simulink model "dfig_group_6_backsave"  (R2019b)
settings: Solver=ode23t  StartTime=0.0  StopTime=100  RelTol=1e-3
undefined symbols (not defined in the file): i, j
libraries: eeGeneralControl x2
settings Model: SimulationMode=accelerator  Creator=aspar  LastModifiedBy=aspar
settings DebuggingCC: UnconnectedInputMsg=none  UnconnectedOutputMsg=none  UnconnectedLineMsg=none
settings ModelReferenceCC: EnableRefExpFcnMdlSchedulingChecks=off
settings RTWCC: Description=Generic Real-Time Target

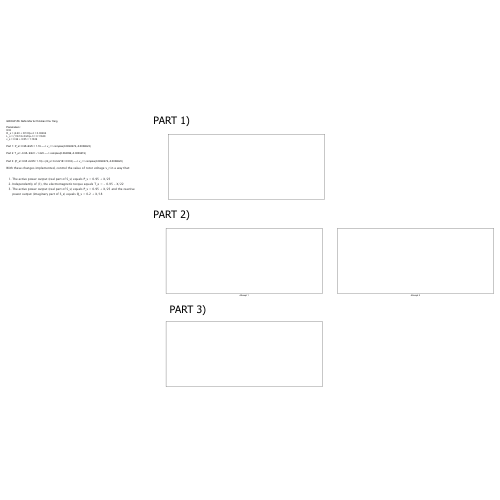
[thumbnail: Simulink's stored preview of the top-level diagram]
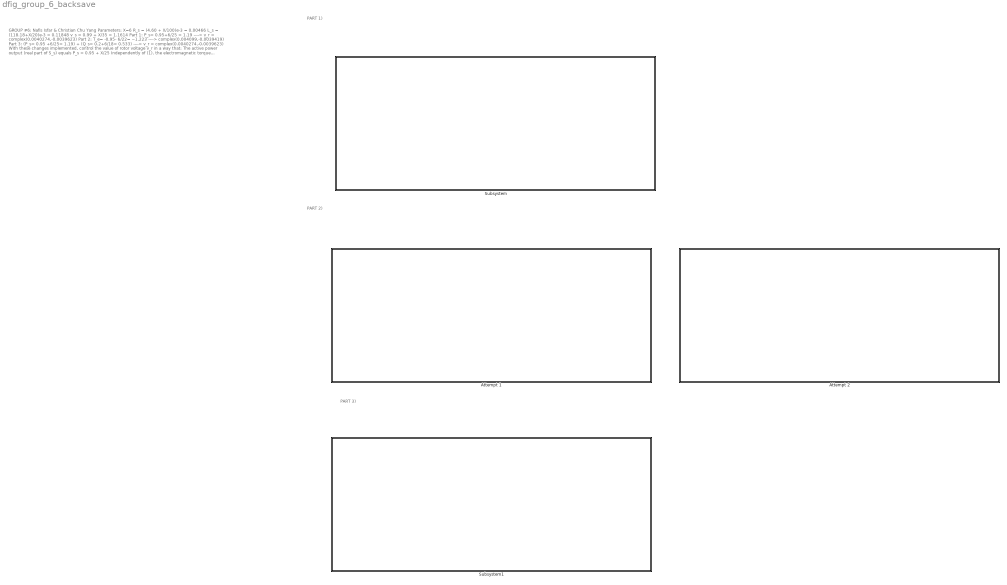
== system dfig_group_6_backsave ==
  note: GROUP #6: Nafis Isfar & Christian Chu Yang
      |
      | Parameters:
      | X=6
      | R_s = (4.60 + X/100)e-3 = 0.00466
      | L_s = (118.18+X/20)e-3 = 0.11848
      | v_s = 0.99 + X/35 = 1.1614
      | Part 1: P_s= 0.95+6/25 = 1.19 ----> v_r = complex(0.0040274,-0.0039623)
      | Part 2: T_e= -0.95- 6/22= −1.223 ----> complex(0.004099,-0.0039419)
      | Part 3: (P_s= 0.95 +6/25= 1.19) + (Q_s= 0.2+6/18= 0.533) ----> v_r = complex(0.0040274,-0.0039623)
      |
      | With these changes implemented, control the value of rotor voltage v_r in a way that:
      | The active power output (real part of S_s) equals P_s = 0.95 + X/25
      | Independently of (1), the electromagnetic torque equals T_e = - 0.95 - X/22
      | The active power output (real part of S_s) equals P_s = 0.95 + X/25 and the reactive power output (imaginary part of S_s) equals Q_s = 0.2 + X/18
  note: PART 1)
  note: PART 2)
  note: PART 3)
  Attempt 1 : Subsystem
  Attempt 2 : Subsystem
  Subsystem : Subsystem
  Subsystem1 : Subsystem

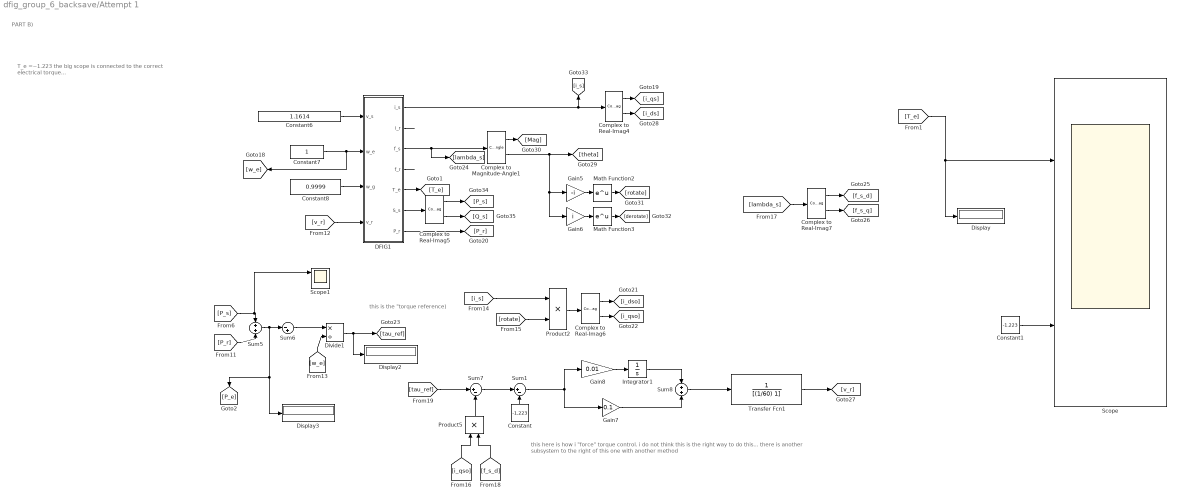
== system dfig_group_6_backsave/Attempt 1 ==
  note: this here is how i "force" torque control. i do not think this is the right way to do this... there is another subsystem to the right of this one with another method
  note: T_e =−1.223
      | the big scope is connected to the correct electrical torque...
  note: this is the "torque reference)
  note: PART B)
  Complex to Magnitude-Angle1 : ComplexToMagnitudeAngle
  Complex to Real-Imag{4..7} (4 alike) : ComplexToRealImag
  Constant : Constant  Value=-1.223
  Constant1 : Constant  Value=-1.223
  Constant6 : Constant  Value=1.1614
  Constant7 : Constant
  Constant8 : Constant  Value=0.9999
  DFIG1 : Subsystem  mask{R_s=4.66e-3, R_r=3.8e-3, L_m=1.99, L_s=118.48e-3}
  Display : Display
  Display2 : Display
  Display3 : Display
  Divide1 : Product  Inputs=*/
  Gain5 : Gain  Gain=-i
  Gain6 : Gain  Gain=i
  Gain7 : Gain  Gain=0.1
  Gain8 : Gain  Gain=0.01
  Integrator1 : Integrator
  Math Function2 : Math  SaturateOnIntegerOverflow=on
  Math Function3 : Math  SaturateOnIntegerOverflow=on
  Product2 : Product
  Product5 : Product
  Scope : Scope  NumInputPorts=2
  Scope1 : Scope  NumInputPorts=3
  Sum1 : Sum  Inputs=|+-
  Sum5 : Sum  Inputs=+|+
  Sum6 : Sum  Inputs=|-+
  Sum7 : Sum  Inputs=|+-
  Sum8 : Sum  Inputs=+|+
  Transfer Fcn1 : TransferFcn  Denominator=[(1/60) 1]
  wires:
  DFIG1/3(f_s) -> Complex to Magnitude-Angle1/1, [lambda_s]
  DFIG1/1(i_s) -> Complex to Real-Imag4/1, [i_s]
  [P_s] -> Sum5/1, Scope1/1
  Sum1/1 -> Gain7/1, Gain8/1
  Transfer Fcn1/1 -> [v_r]
  Sum6/1 -> Divide1/1
  [rotate] -> Product2/2
  Sum8/1 -> Transfer Fcn1/1
  DFIG1/4(f_r) -> ?
  Complex to Magnitude-Angle1/2 -> [theta], Gain5/1, Gain6/1
  Gain7/1 -> Sum8/2
  [i_qso] -> Product5/1
  DFIG1/7(P_r) -> [P_r]
  Gain8/1 -> Integrator1/1
  [f_s_d] -> Product5/2
  Complex to Real-Imag6/2 -> [i_qso]
  Math Function3/1 -> [derotate]
  Divide1/1 -> [tau_ref], Display2/1
  [tau_ref] -> Sum7/1
  Complex to Real-Imag7/1 -> [f_s_d]
  Constant6/1 -> DFIG1/1(v_s)
  [lambda_s] -> Complex to Real-Imag7/1
  Gain6/1 -> Math Function3/1
  Complex to Real-Imag4/2 -> [i_ds]
  [i_s] -> Product2/1
  [w_e] -> Divide1/2
  Complex to Real-Imag5/1 -> [P_s]
  Complex to Real-Imag7/2 -> [f_s_q]
  Product5/1 -> Sum7/2
  Product2/1 -> Complex to Real-Imag6/1
  Complex to Real-Imag6/1 -> [i_dso]
  Integrator1/1 -> Sum8/1
  Gain5/1 -> Math Function2/1
  Sum5/1 -> [P_e], Display3/1, Sum6/1
  DFIG1/6(S_s) -> Complex to Real-Imag5/1
  Math Function2/1 -> [rotate]
  Complex to Real-Imag5/2 -> [Q_s]
  Complex to Real-Imag4/1 -> [i_qs]
  Constant8/1 -> DFIG1/3(w_g)
  Complex to Magnitude-Angle1/1 -> [Mag]
  Constant7/1 -> [w_e], DFIG1/2(w_e)
  [v_r] -> DFIG1/4(v_r)
  DFIG1/2(i_r) -> ?
  [P_r] -> Sum5/2
  DFIG1/5(T_e) -> [T_e]
  [T_e] -> Display/1, Scope/1
  Sum7/1 -> Sum1/1
  Constant/1 -> Sum1/2
  Constant1/1 -> Scope/2

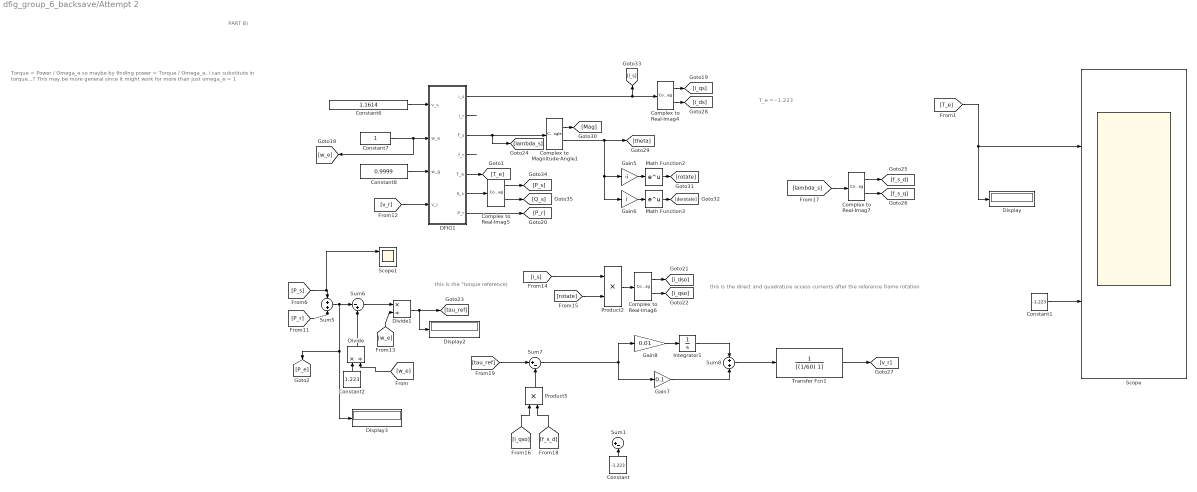
== system dfig_group_6_backsave/Attempt 2 ==
  note: Torque = Power / Omega_e
      | so maybe by finding power = Torque / Omega_e, i can substitute in torque...?
      | This may be more general since it might work for more than just omega_e = 1
  note: T_e =−1.223
  note: this is the direct and quadrature access currents after the reference frame rotation
  note: this is the "torque reference)
  note: PART B)
  Complex to Magnitude-Angle1 : ComplexToMagnitudeAngle
  Complex to Real-Imag{4..7} (4 alike) : ComplexToRealImag
  Constant : Constant  Value=-1.223
  Constant1 : Constant  Value=-1.223
  Constant2 : Constant  Value=1.223
  Constant6 : Constant  Value=1.1614
  Constant7 : Constant
  Constant8 : Constant  Value=0.9999
  DFIG1 : Subsystem  mask{R_s=4.66e-3, R_r=3.8e-3, L_m=1.99, L_s=118.48e-3}
  Display : Display
  Display2 : Display
  Display3 : Display
  Divide : Product  Inputs=*/
  Divide1 : Product  Inputs=*/
  Gain5 : Gain  Gain=-i
  Gain6 : Gain  Gain=i
  Gain7 : Gain  Gain=0.1
  Gain8 : Gain  Gain=0.01
  Integrator1 : Integrator
  Math Function2 : Math  SaturateOnIntegerOverflow=on
  Math Function3 : Math  SaturateOnIntegerOverflow=on
  Product2 : Product
  Product5 : Product
  Scope : Scope  NumInputPorts=2
  Scope1 : Scope  NumInputPorts=3
  Sum1 : Sum  Inputs=|+-
  Sum5 : Sum  Inputs=+|+
  Sum6 : Sum  Inputs=|-+
  Sum7 : Sum  Inputs=|+-
  Sum8 : Sum  Inputs=+|+
  Transfer Fcn1 : TransferFcn  Denominator=[(1/60) 1]
  wires:
  DFIG1/3(f_s) -> Complex to Magnitude-Angle1/1, [lambda_s]
  DFIG1/1(i_s) -> Complex to Real-Imag4/1, [i_s]
  [P_s] -> Sum5/1, Scope1/1
  Sum7/1 -> Gain7/1, Gain8/1
  Transfer Fcn1/1 -> [v_r]
  Sum6/1 -> Divide1/1
  [rotate] -> Product2/2
  Sum8/1 -> Transfer Fcn1/1
  DFIG1/4(f_r) -> ?
  Complex to Magnitude-Angle1/2 -> [theta], Gain5/1, Gain6/1
  Gain7/1 -> Sum8/2
  [i_qso] -> Product5/1
  DFIG1/7(P_r) -> [P_r]
  Gain8/1 -> Integrator1/1
  [f_s_d] -> Product5/2
  Complex to Real-Imag6/2 -> [i_qso]
  Math Function3/1 -> [derotate]
  Divide1/1 -> [tau_ref], Display2/1
  [tau_ref] -> Sum7/1
  Complex to Real-Imag7/1 -> [f_s_d]
  Constant6/1 -> DFIG1/1(v_s)
  [lambda_s] -> Complex to Real-Imag7/1
  Gain6/1 -> Math Function3/1
  Complex to Real-Imag4/2 -> [i_ds]
  [i_s] -> Product2/1
  [w_e] -> Divide1/2
  Complex to Real-Imag5/1 -> [P_s]
  Complex to Real-Imag7/2 -> [f_s_q]
  Product5/1 -> Sum7/2
  Product2/1 -> Complex to Real-Imag6/1
  Complex to Real-Imag6/1 -> [i_dso]
  Integrator1/1 -> Sum8/1
  Gain5/1 -> Math Function2/1
  Sum5/1 -> [P_e], Display3/1, Sum6/1
  DFIG1/6(S_s) -> Complex to Real-Imag5/1
  Math Function2/1 -> [rotate]
  Complex to Real-Imag5/2 -> [Q_s]
  Complex to Real-Imag4/1 -> [i_qs]
  Constant8/1 -> DFIG1/3(w_g)
  Complex to Magnitude-Angle1/1 -> [Mag]
  Constant7/1 -> [w_e], DFIG1/2(w_e)
  [v_r] -> DFIG1/4(v_r)
  DFIG1/2(i_r) -> ?
  [P_r] -> Sum5/2
  DFIG1/5(T_e) -> [T_e]
  [T_e] -> Display/1, Scope/1
  Constant1/1 -> Scope/2
  Constant/1 -> Sum1/2
  Divide/1 -> Sum6/2
  Constant2/1 -> Divide/1
  [w_e] -> Divide/2

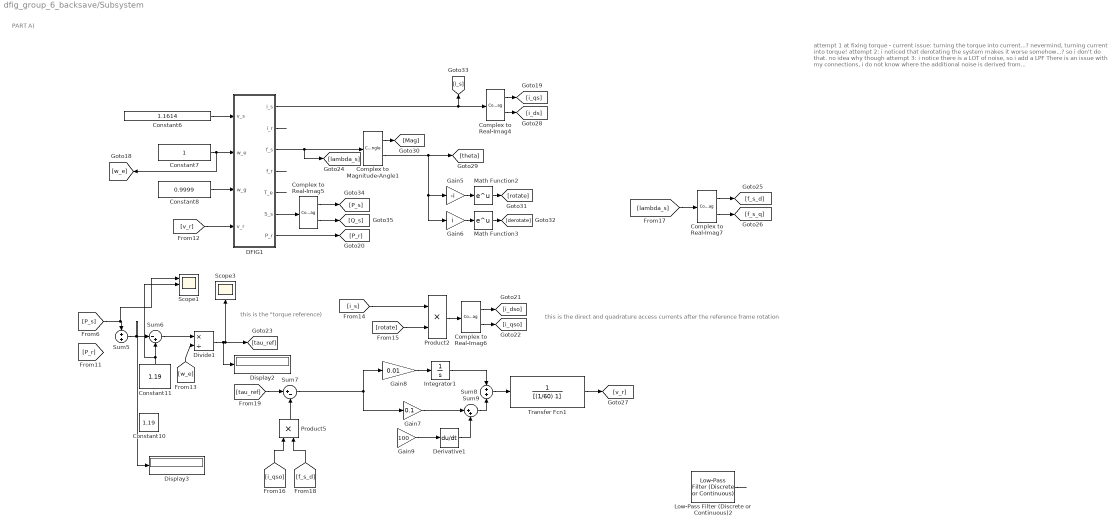
== system dfig_group_6_backsave/Subsystem ==
  note: this is the direct and quadrature access currents after the reference frame rotation
  note: attempt 1 at fixing torque - current issue: turning the torque into current...? nevermind, turning current into torque!
      |
      | attempt 2: i noticed that derotating the system makes it worse somehow...? so i don't do that. no idea why though
      |
      | attempt 3: i notice there is a LOT of noise, so i add a LPF
      |
      | There is an issue with my connections, i do not know where the additional noise is derived from...
  note: this is the "torque reference)
  note: PART A)
  Complex to Magnitude-Angle1 : ComplexToMagnitudeAngle
  Complex to Real-Imag{4..7} (4 alike) : ComplexToRealImag
  Constant10 : Constant  Value=1.19
  Constant11 : Constant  Value=1.19
  Constant6 : Constant  Value=1.1614
  Constant7 : Constant
  Constant8 : Constant  Value=0.9999
  DFIG1 : Subsystem  mask{R_s=4.66e-3, R_r=3.8e-3, L_m=1.99, L_s=118.48e-3}
  Derivative1 : Derivative
  Display2 : Display
  Display3 : Display
  Divide1 : Product  Inputs=*/
  Gain5 : Gain  Gain=-i
  Gain6 : Gain  Gain=i
  Gain7 : Gain  Gain=0.1
  Gain8 : Gain  Gain=0.01
  Gain9 : Gain  Gain=100
  Integrator1 : Integrator
  Low-Pass Filter (Discrete or Continuous)2 : eeGeneralControl/Low-Pass Filter (Discrete or Continuous)  K=1  T=1/60  B=inf  A=-inf  init_option=Inherited from block input  x0=0  Ts=-1
  Math Function2 : Math  SaturateOnIntegerOverflow=on
  Math Function3 : Math  SaturateOnIntegerOverflow=on
  Product2 : Product
  Product5 : Product
  Scope1 : Scope  NumInputPorts=3
  Scope3 : Scope
  Sum5 : Sum  Inputs=+|+
  Sum6 : Sum  Inputs=|-+
  Sum7 : Sum  Inputs=|+-
  Sum8 : Sum  Inputs=+|+
  Sum9 : Sum  Inputs=|++
  Transfer Fcn1 : TransferFcn  Denominator=[(1/60) 1]
  wires:
  DFIG1/3(f_s) -> Complex to Magnitude-Angle1/1, [lambda_s]
  DFIG1/1(i_s) -> Complex to Real-Imag4/1, [i_s]
  [P_s] -> Sum5/1, Scope1/1
  Gain9/1 -> Derivative1/1
  Sum7/1 -> Gain7/1, Gain8/1
  Transfer Fcn1/1 -> [v_r]
  Gain7/1 -> Sum9/1
  Sum6/1 -> Divide1/1
  [rotate] -> Product2/2
  Sum8/1 -> Transfer Fcn1/1
  DFIG1/4(f_r) -> ?
  Complex to Magnitude-Angle1/2 -> [theta], Gain5/1, Gain6/1
  Sum9/1 -> Sum8/2
  Derivative1/1 -> Sum9/2
  [i_qso] -> Product5/1
  DFIG1/7(P_r) -> [P_r]
  Gain8/1 -> Integrator1/1
  ? -> Gain9/1
  [f_s_d] -> Product5/2
  Complex to Real-Imag6/2 -> [i_qso]
  Math Function3/1 -> [derotate]
  DFIG1/5(T_e) -> ?
  Divide1/1 -> [tau_ref], Scope3/1, Display2/1
  [tau_ref] -> Sum7/1
  Constant11/1 -> Sum6/2, Scope1/2
  Complex to Real-Imag7/1 -> [f_s_d]
  Constant6/1 -> DFIG1/1(v_s)
  [lambda_s] -> Complex to Real-Imag7/1
  Gain6/1 -> Math Function3/1
  ? -> Low-Pass Filter (Discrete or Continuous)2/1
  Complex to Real-Imag4/2 -> [i_ds]
  [i_s] -> Product2/1
  [w_e] -> Divide1/2
  Complex to Real-Imag5/1 -> [P_s]
  Complex to Real-Imag7/2 -> [f_s_q]
  Product5/1 -> Sum7/2
  Product2/1 -> Complex to Real-Imag6/1
  Complex to Real-Imag6/1 -> [i_dso]
  Integrator1/1 -> Sum8/1
  Gain5/1 -> Math Function2/1
  Sum5/1 -> Sum6/1, Display3/1
  DFIG1/6(S_s) -> Complex to Real-Imag5/1
  Math Function2/1 -> [rotate]
  Complex to Real-Imag5/2 -> [Q_s]
  Complex to Real-Imag4/1 -> [i_qs]
  Constant8/1 -> DFIG1/3(w_g)
  Complex to Magnitude-Angle1/1 -> [Mag]
  Constant7/1 -> DFIG1/2(w_e), [w_e]
  [v_r] -> DFIG1/4(v_r)
  DFIG1/2(i_r) -> ?
  Low-Pass Filter (Discrete or Continuous)2/1 -> ?

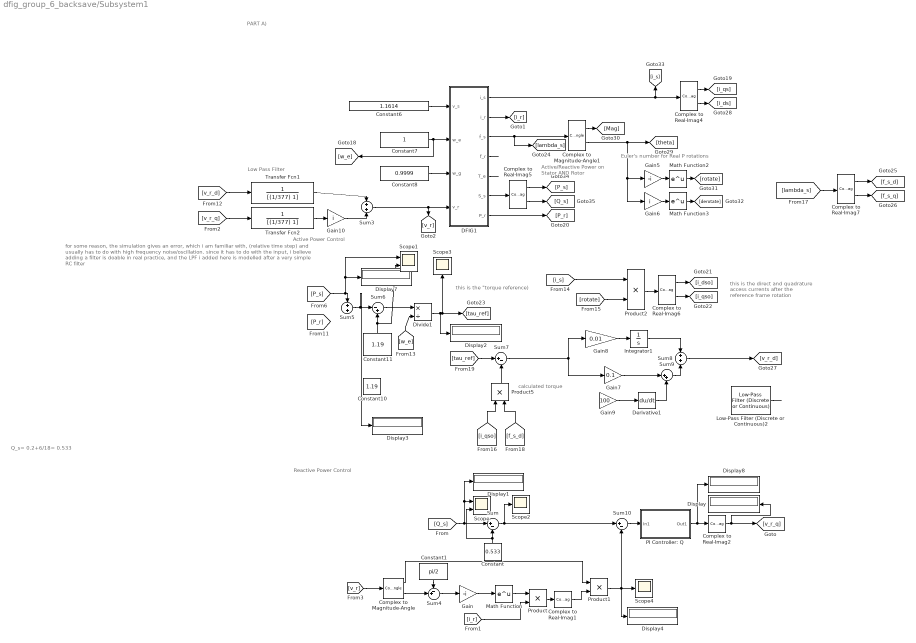
== system dfig_group_6_backsave/Subsystem1 ==
  note: calculated torque
  note: Euler's number for Real P rotations
  note: Active/Reactive
      | Power on
      | Stator AND Rotor
  note: Reactive Power Control
  note: Low Pass Filter
  note: for some reason, the simulation gives an error,
      | which i am familiar with, (relative time step)
      | and usually has to do with high frequency
      | noise/oscillation. since it has to do with the input,
      | i believe adding a filter is doable in real practice,
      | and the LPF i added here is modelled after a
      | very simple RC filter
  note: Q_s= 0.2+6/18= 0.533
  note: Active Power
      | Control
  note: this is the direct and quadrature access currents after the reference frame rotation
  note: this is the "torque reference)
  note: PART A)
  Complex to Magnitude-Angle : ComplexToMagnitudeAngle
  Complex to Magnitude-Angle1 : ComplexToMagnitudeAngle
  Complex to Real-Imag1 : ComplexToRealImag  Output=Real
  Complex to Real-Imag2 : ComplexToRealImag  Output=Real
  Complex to Real-Imag{4..7} (4 alike) : ComplexToRealImag
  Constant : Constant  Value=0.533
  Constant1 : Constant  Value=pi/2
  Constant10 : Constant  Value=1.19
  Constant11 : Constant  Value=1.19
  Constant6 : Constant  Value=1.1614
  Constant7 : Constant
  Constant8 : Constant  Value=0.9999
  DFIG1 : Subsystem  mask{R_s=4.66e-3, R_r=3.8e-3, L_m=1.99, L_s=118.48e-3}
  Derivative1 : Derivative
  Display{,1..4,7..8} (7 alike) : Display
  Divide1 : Product  Inputs=*/
  Gain : Gain  Gain=-i
  Gain10 : Gain  Gain=i
  Gain5 : Gain  Gain=-i
  Gain6 : Gain  Gain=i
  Gain7 : Gain  Gain=0.1
  Gain8 : Gain  Gain=0.01
  Gain9 : Gain  Gain=100
  Integrator1 : Integrator
  Low-Pass Filter (Discrete or Continuous)2 : eeGeneralControl/Low-Pass Filter (Discrete or Continuous)  K=1  T=1/60  B=inf  A=-inf  init_option=Inherited from block input  x0=0  Ts=-1
  Math Function : Math  SaturateOnIntegerOverflow=on
  Math Function2 : Math  SaturateOnIntegerOverflow=on
  Math Function3 : Math  SaturateOnIntegerOverflow=on
  PI Controller: Q : Subsystem
  Product{,1..2,5} (4 alike) : Product
  Scope : Scope  NumInputPorts=2
  Scope1 : Scope  NumInputPorts=2
  Scope2 : Scope
  Scope3 : Scope
  Scope4 : Scope
  Sum : Sum  Inputs=|+-
  Sum10 : Sum  Inputs=|+-
  Sum3 : Sum  Inputs=+|+
  Sum4 : Sum  Inputs=-+|
  Sum5 : Sum  Inputs=+|+
  Sum6 : Sum  Inputs=|-+
  Sum7 : Sum  Inputs=|+-
  Sum8 : Sum  Inputs=+|+
  Sum9 : Sum  Inputs=|++
  Transfer Fcn1 : TransferFcn  Denominator=[(1/377) 1]
  Transfer Fcn2 : TransferFcn  Denominator=[(1/377) 1]
  wires:
  DFIG1/3(f_s) -> Complex to Magnitude-Angle1/1, [lambda_s]
  DFIG1/1(i_s) -> Complex to Real-Imag4/1, [i_s]
  [P_s] -> Sum5/1, Display7/1, Scope1/1
  Gain9/1 -> Derivative1/1
  Sum7/1 -> Gain7/1, Gain8/1
  Sum8/1 -> [v_r_d]
  Gain7/1 -> Sum9/1
  Sum6/1 -> Divide1/1
  [rotate] -> Product2/2
  DFIG1/4(f_r) -> ?
  Complex to Magnitude-Angle1/2 -> [theta], Gain5/1, Gain6/1
  Sum9/1 -> Sum8/2
  Derivative1/1 -> Sum9/2
  [i_qso] -> Product5/1
  DFIG1/7(P_r) -> [P_r]
  Gain8/1 -> Integrator1/1
  ? -> Gain9/1
  [f_s_d] -> Product5/2
  Complex to Real-Imag6/2 -> [i_qso]
  Math Function3/1 -> [derotate]
  DFIG1/5(T_e) -> ?
  Divide1/1 -> [tau_ref], Scope3/1, Display2/1
  [tau_ref] -> Sum7/1
  Constant11/1 -> Sum6/2, Scope1/2
  Complex to Real-Imag7/1 -> [f_s_d]
  Constant6/1 -> DFIG1/1(v_s)
  [lambda_s] -> Complex to Real-Imag7/1
  Gain6/1 -> Math Function3/1
  ? -> Low-Pass Filter (Discrete or Continuous)2/1
  Complex to Real-Imag4/2 -> [i_ds]
  [i_s] -> Product2/1
  [w_e] -> Divide1/2
  Complex to Real-Imag5/1 -> [P_s]
  Complex to Real-Imag7/2 -> [f_s_q]
  Product5/1 -> Sum7/2
  Product2/1 -> Complex to Real-Imag6/1
  Complex to Real-Imag6/1 -> [i_dso]
  Integrator1/1 -> Sum8/1
  Gain5/1 -> Math Function2/1
  Sum5/1 -> Sum6/1, Display3/1
  DFIG1/6(S_s) -> Complex to Real-Imag5/1
  Math Function2/1 -> [rotate]
  Complex to Real-Imag5/2 -> [Q_s]
  Complex to Real-Imag4/1 -> [i_qs]
  Constant8/1 -> DFIG1/3(w_g)
  Complex to Magnitude-Angle1/1 -> [Mag]
  Constant7/1 -> DFIG1/2(w_e), [w_e]
  DFIG1/2(i_r) -> [i_r]
  Low-Pass Filter (Discrete or Continuous)2/1 -> ?
  [Q_s] -> Display1/1, Scope/1, Sum/1
  Constant/1 -> Scope/2, Sum/2
  Sum3/1 -> [v_r], DFIG1/4(v_r)
  [v_r] -> Complex to Magnitude-Angle/1
  Constant1/1 -> Sum4/1
  Sum4/1 -> Gain/1
  Gain/1 -> Math Function/1
  Math Function/1 -> Product/1
  [i_r] -> Product/2
  Complex to Magnitude-Angle/1 -> Product1/1
  Sum/1 -> Sum10/1, Scope2/1
  Product1/1 -> Sum10/2, Display4/1, Scope4/1
  Complex to Magnitude-Angle/2 -> Sum4/2
  Product/1 -> Complex to Real-Imag1/1
  Complex to Real-Imag1/1 -> Product1/2
  [v_r_d] -> Transfer Fcn1/1
  Transfer Fcn2/1 -> Gain10/1
  Transfer Fcn1/1 -> Sum3/1
  Gain10/1 -> Sum3/2
  [v_r_q] -> Transfer Fcn2/1
  Complex to Real-Imag2/1 -> [v_r_q], Display/1
  PI Controller: Q/1(Out1) -> Display8/1, Complex to Real-Imag2/1
  Sum10/1 -> PI Controller: Q/1(In1)

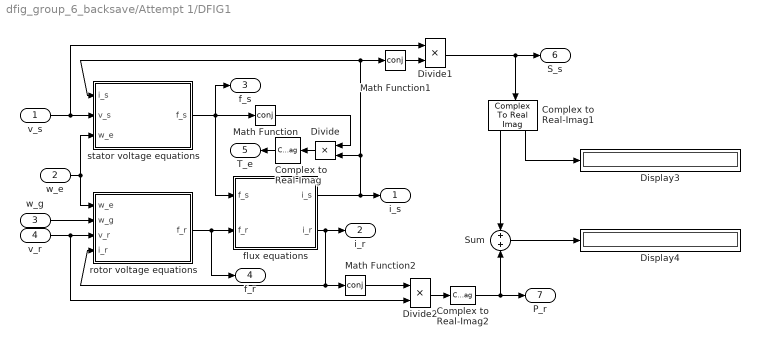
== system dfig_group_6_backsave/Attempt 1/DFIG1 ==
  v_s : Inport
  w_e : Inport  Port=2
  w_g : Inport  Port=3
  v_r : Inport  Port=4
  Complex to Real-Imag : ComplexToRealImag  Output=Imag
  Complex to Real-Imag1 : ComplexToRealImag
  Complex to Real-Imag2 : ComplexToRealImag  Output=Real
  Display3 : Display
  Display4 : Display
  Divide : Product  Inputs=**
  Divide1 : Product  Inputs=**
  Divide2 : Product  Inputs=**
  Math Function : Math  Operator=conj  SignedPower=on  SaturateOnIntegerOverflow=on
  Math Function1 : Math  Operator=conj  SignedPower=on  SaturateOnIntegerOverflow=on
  Math Function2 : Math  Operator=conj  SignedPower=on  SaturateOnIntegerOverflow=on
  Sum : Sum
  flux equations : Subsystem
  rotor voltage equations : Subsystem
  stator voltage equations : Subsystem
  i_s : Outport
  i_r : Outport  Port=2
  f_s : Outport  Port=3
  f_r : Outport  Port=4
  T_e : Outport  Port=5
  S_s : Outport  Port=6
  P_r : Outport  Port=7
  wires:
  Complex to Real-Imag2/1 -> Sum/2, P_r/1
  Math Function2/1 -> Divide2/1
  stator voltage equations/1(f_s) -> flux equations/1(f_s), f_s/1, Math Function/1
  Math Function/1 -> Divide/1
  Divide2/1 -> Complex to Real-Imag2/1
  Divide1/1 -> Complex to Real-Imag1/1, S_s/1
  Math Function1/1 -> Divide1/2
  Complex to Real-Imag/1 -> T_e/1
  Divide/1 -> Complex to Real-Imag/1
  rotor voltage equations/1(f_r) -> flux equations/2(f_r), f_r/1
  flux equations/2(i_r) -> Math Function2/1, rotor voltage equations/4(i_r), i_r/1
  flux equations/1(i_s) -> Divide/2, stator voltage equations/1(i_s), Math Function1/1, i_s/1
  v_r/1 -> rotor voltage equations/3(v_r), Divide2/2
  w_e/1 -> rotor voltage equations/1(w_e), stator voltage equations/3(w_e)
  v_s/1 -> Divide1/1, stator voltage equations/2(v_s)
  w_g/1 -> rotor voltage equations/2(w_g)
  Sum/1 -> Display4/1
  Complex to Real-Imag1/1 -> Sum/1
  Complex to Real-Imag1/2 -> Display3/1

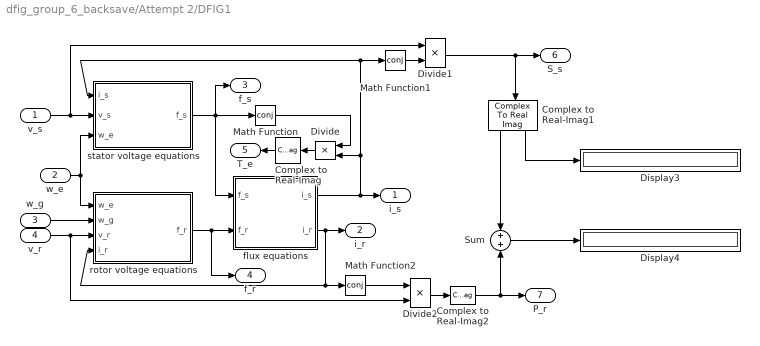
== system dfig_group_6_backsave/Attempt 2/DFIG1 ==
  v_s : Inport
  w_e : Inport  Port=2
  w_g : Inport  Port=3
  v_r : Inport  Port=4
  Complex to Real-Imag : ComplexToRealImag  Output=Imag
  Complex to Real-Imag1 : ComplexToRealImag
  Complex to Real-Imag2 : ComplexToRealImag  Output=Real
  Display3 : Display
  Display4 : Display
  Divide : Product  Inputs=**
  Divide1 : Product  Inputs=**
  Divide2 : Product  Inputs=**
  Math Function : Math  Operator=conj  SignedPower=on  SaturateOnIntegerOverflow=on
  Math Function1 : Math  Operator=conj  SignedPower=on  SaturateOnIntegerOverflow=on
  Math Function2 : Math  Operator=conj  SignedPower=on  SaturateOnIntegerOverflow=on
  Sum : Sum
  flux equations : Subsystem
  rotor voltage equations : Subsystem
  stator voltage equations : Subsystem
  i_s : Outport
  i_r : Outport  Port=2
  f_s : Outport  Port=3
  f_r : Outport  Port=4
  T_e : Outport  Port=5
  S_s : Outport  Port=6
  P_r : Outport  Port=7
  wires:
  Complex to Real-Imag2/1 -> Sum/2, P_r/1
  Math Function2/1 -> Divide2/1
  stator voltage equations/1(f_s) -> flux equations/1(f_s), f_s/1, Math Function/1
  Math Function/1 -> Divide/1
  Divide2/1 -> Complex to Real-Imag2/1
  Divide1/1 -> Complex to Real-Imag1/1, S_s/1
  Math Function1/1 -> Divide1/2
  Complex to Real-Imag/1 -> T_e/1
  Divide/1 -> Complex to Real-Imag/1
  rotor voltage equations/1(f_r) -> flux equations/2(f_r), f_r/1
  flux equations/2(i_r) -> Math Function2/1, rotor voltage equations/4(i_r), i_r/1
  flux equations/1(i_s) -> Divide/2, stator voltage equations/1(i_s), Math Function1/1, i_s/1
  v_r/1 -> rotor voltage equations/3(v_r), Divide2/2
  w_e/1 -> rotor voltage equations/1(w_e), stator voltage equations/3(w_e)
  v_s/1 -> Divide1/1, stator voltage equations/2(v_s)
  w_g/1 -> rotor voltage equations/2(w_g)
  Sum/1 -> Display4/1
  Complex to Real-Imag1/1 -> Sum/1
  Complex to Real-Imag1/2 -> Display3/1

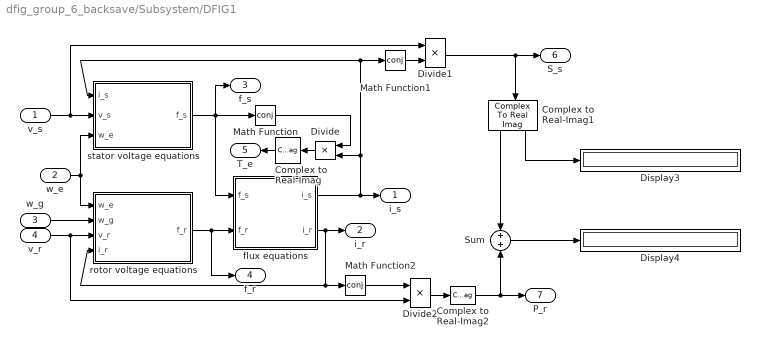
== system dfig_group_6_backsave/Subsystem/DFIG1 ==
  v_s : Inport
  w_e : Inport  Port=2
  w_g : Inport  Port=3
  v_r : Inport  Port=4
  Complex to Real-Imag : ComplexToRealImag  Output=Imag
  Complex to Real-Imag1 : ComplexToRealImag
  Complex to Real-Imag2 : ComplexToRealImag  Output=Real
  Display3 : Display
  Display4 : Display
  Divide : Product  Inputs=**
  Divide1 : Product  Inputs=**
  Divide2 : Product  Inputs=**
  Math Function : Math  Operator=conj  SignedPower=on  SaturateOnIntegerOverflow=on
  Math Function1 : Math  Operator=conj  SignedPower=on  SaturateOnIntegerOverflow=on
  Math Function2 : Math  Operator=conj  SignedPower=on  SaturateOnIntegerOverflow=on
  Sum : Sum
  flux equations : Subsystem
  rotor voltage equations : Subsystem
  stator voltage equations : Subsystem
  i_s : Outport
  i_r : Outport  Port=2
  f_s : Outport  Port=3
  f_r : Outport  Port=4
  T_e : Outport  Port=5
  S_s : Outport  Port=6
  P_r : Outport  Port=7
  wires:
  Complex to Real-Imag2/1 -> Sum/2, P_r/1
  Math Function2/1 -> Divide2/1
  stator voltage equations/1(f_s) -> flux equations/1(f_s), f_s/1, Math Function/1
  Math Function/1 -> Divide/1
  Divide2/1 -> Complex to Real-Imag2/1
  Divide1/1 -> Complex to Real-Imag1/1, S_s/1
  Math Function1/1 -> Divide1/2
  Complex to Real-Imag/1 -> T_e/1
  Divide/1 -> Complex to Real-Imag/1
  rotor voltage equations/1(f_r) -> flux equations/2(f_r), f_r/1
  flux equations/2(i_r) -> Math Function2/1, rotor voltage equations/4(i_r), i_r/1
  flux equations/1(i_s) -> Divide/2, stator voltage equations/1(i_s), Math Function1/1, i_s/1
  v_r/1 -> rotor voltage equations/3(v_r), Divide2/2
  w_e/1 -> rotor voltage equations/1(w_e), stator voltage equations/3(w_e)
  v_s/1 -> Divide1/1, stator voltage equations/2(v_s)
  w_g/1 -> rotor voltage equations/2(w_g)
  Sum/1 -> Display4/1
  Complex to Real-Imag1/1 -> Sum/1
  Complex to Real-Imag1/2 -> Display3/1

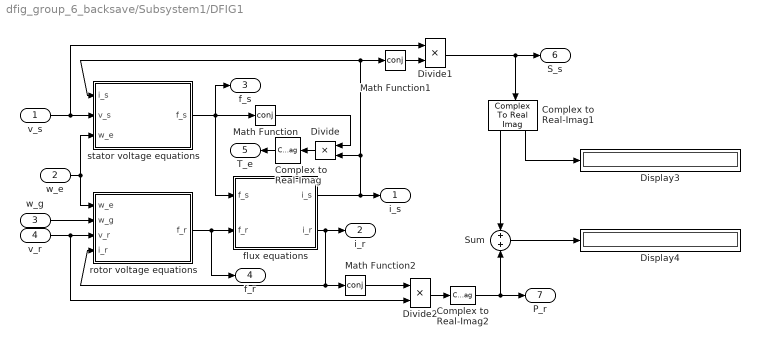
== system dfig_group_6_backsave/Subsystem1/DFIG1 ==
  v_s : Inport
  w_e : Inport  Port=2
  w_g : Inport  Port=3
  v_r : Inport  Port=4
  Complex to Real-Imag : ComplexToRealImag  Output=Imag
  Complex to Real-Imag1 : ComplexToRealImag
  Complex to Real-Imag2 : ComplexToRealImag  Output=Real
  Display3 : Display
  Display4 : Display
  Divide : Product  Inputs=**
  Divide1 : Product  Inputs=**
  Divide2 : Product  Inputs=**
  Math Function : Math  Operator=conj  SignedPower=on  SaturateOnIntegerOverflow=on
  Math Function1 : Math  Operator=conj  SignedPower=on  SaturateOnIntegerOverflow=on
  Math Function2 : Math  Operator=conj  SignedPower=on  SaturateOnIntegerOverflow=on
  Sum : Sum
  flux equations : Subsystem
  rotor voltage equations : Subsystem
  stator voltage equations : Subsystem
  i_s : Outport
  i_r : Outport  Port=2
  f_s : Outport  Port=3
  f_r : Outport  Port=4
  T_e : Outport  Port=5
  S_s : Outport  Port=6
  P_r : Outport  Port=7
  wires:
  Complex to Real-Imag2/1 -> Sum/2, P_r/1
  Math Function2/1 -> Divide2/1
  stator voltage equations/1(f_s) -> flux equations/1(f_s), f_s/1, Math Function/1
  Math Function/1 -> Divide/1
  Divide2/1 -> Complex to Real-Imag2/1
  Divide1/1 -> Complex to Real-Imag1/1, S_s/1
  Math Function1/1 -> Divide1/2
  Complex to Real-Imag/1 -> T_e/1
  Divide/1 -> Complex to Real-Imag/1
  rotor voltage equations/1(f_r) -> flux equations/2(f_r), f_r/1
  flux equations/2(i_r) -> Math Function2/1, rotor voltage equations/4(i_r), i_r/1
  flux equations/1(i_s) -> Divide/2, stator voltage equations/1(i_s), Math Function1/1, i_s/1
  v_r/1 -> rotor voltage equations/3(v_r), Divide2/2
  w_e/1 -> rotor voltage equations/1(w_e), stator voltage equations/3(w_e)
  v_s/1 -> Divide1/1, stator voltage equations/2(v_s)
  w_g/1 -> rotor voltage equations/2(w_g)
  Sum/1 -> Display4/1
  Complex to Real-Imag1/1 -> Sum/1
  Complex to Real-Imag1/2 -> Display3/1

== system dfig_group_6_backsave/Subsystem1/PI Controller: Q ==
  In1 : Inport
  Complex to Real-Imag : ComplexToRealImag
  Gain1 : Gain  Gain=0.1
  Gain2 : Gain  Gain=0.01
  Gain3 : Gain  Gain=i
  Integrator2 : Integrator
  Integrator3 : Integrator
  Sum1 : Sum  Inputs=+|+
  Sum11 : Sum  Inputs=+|+
  Out1 : Outport
  wires:
  Gain1/1 -> Sum1/2
  Complex to Real-Imag/2 -> Integrator2/1
  Gain2/1 -> Complex to Real-Imag/1
  In1/1 -> Gain2/1, Gain1/1
  Sum11/1 -> Sum1/1
  Gain3/1 -> Sum11/2
  Integrator2/1 -> Gain3/1
  Complex to Real-Imag/1 -> Integrator3/1
  Integrator3/1 -> Sum11/1
  Sum1/1 -> Out1/1

== system dfig_group_6_backsave/Attempt 1/DFIG1/flux equations ==
  f_s : Inport
  f_r : Inport  Port=2
  Gain5 : Gain  Gain=1/L_s
  Gain7 : Gain  Gain=1/L_m
  Sum1 : Sum  Inputs=|+-
  Sum5 : Sum  Inputs=-+|
  i_s : Outport
  i_r : Outport  Port=2
  wires:
  Sum1/1 -> i_s/1
  Gain7/1 -> Sum1/1
  Sum5/1 -> Gain5/1
  f_r/1 -> Sum5/2
  Gain5/1 -> Sum1/2, i_r/1
  f_s/1 -> Sum5/1, Gain7/1

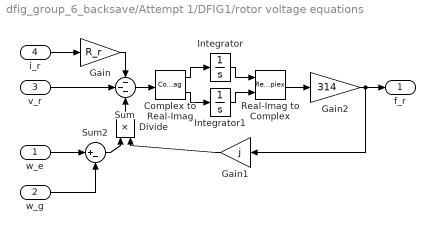
== system dfig_group_6_backsave/Attempt 1/DFIG1/rotor voltage equations ==
  w_e : Inport
  w_g : Inport  Port=2
  v_r : Inport  Port=3
  i_r : Inport  Port=4
  Complex to Real-Imag : ComplexToRealImag
  Divide : Product  Inputs=**
  Gain : Gain  Gain=R_r
  Gain1 : Gain  Gain=j
  Gain2 : Gain  Gain=314
  Integrator : Integrator
  Integrator1 : Integrator
  Real-Imag to Complex : RealImagToComplex
  Sum : Sum  Inputs=---
  Sum2 : Sum  Inputs=|+-
  f_r : Outport
  wires:
  Gain2/1 -> Gain1/1, f_r/1
  Gain1/1 -> Divide/2
  Complex to Real-Imag/2 -> Integrator1/1
  Complex to Real-Imag/1 -> Integrator/1
  Sum/1 -> Complex to Real-Imag/1
  w_g/1 -> Sum2/2
  w_e/1 -> Sum2/1
  Gain/1 -> Sum/1
  v_r/1 -> Sum/2
  i_r/1 -> Gain/1
  Real-Imag to Complex/1 -> Gain2/1
  Sum2/1 -> Divide/1
  Divide/1 -> Sum/3
  Integrator1/1 -> Real-Imag to Complex/2
  Integrator/1 -> Real-Imag to Complex/1

== system dfig_group_6_backsave/Attempt 1/DFIG1/stator voltage equations ==
  i_s : Inport
  v_s : Inport  Port=2
  w_e : Inport  Port=3
  Complex to Real-Imag : ComplexToRealImag
  Divide : Product  Inputs=**
  Gain : Gain  Gain=R_s
  Gain1 : Gain  Gain=j
  Gain2 : Gain  Gain=314
  Integrator : Integrator
  Integrator1 : Integrator
  Real-Imag to Complex : RealImagToComplex
  Sum : Sum  Inputs=---
  f_s : Outport
  wires:
  Gain2/1 -> Gain1/1, f_s/1
  Gain1/1 -> Divide/2
  Complex to Real-Imag/2 -> Integrator1/1
  Complex to Real-Imag/1 -> Integrator/1
  Sum/1 -> Complex to Real-Imag/1
  v_s/1 -> Sum/2
  Gain/1 -> Sum/1
  i_s/1 -> Gain/1
  Real-Imag to Complex/1 -> Gain2/1
  w_e/1 -> Divide/1
  Divide/1 -> Sum/3
  Integrator1/1 -> Real-Imag to Complex/2
  Integrator/1 -> Real-Imag to Complex/1

== system dfig_group_6_backsave/Attempt 2/DFIG1/flux equations ==
  f_s : Inport
  f_r : Inport  Port=2
  Gain5 : Gain  Gain=1/L_s
  Gain7 : Gain  Gain=1/L_m
  Sum1 : Sum  Inputs=|+-
  Sum5 : Sum  Inputs=-+|
  i_s : Outport
  i_r : Outport  Port=2
  wires:
  Sum1/1 -> i_s/1
  Gain7/1 -> Sum1/1
  Sum5/1 -> Gain5/1
  f_r/1 -> Sum5/2
  Gain5/1 -> Sum1/2, i_r/1
  f_s/1 -> Sum5/1, Gain7/1

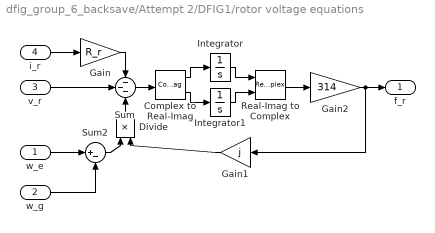
== system dfig_group_6_backsave/Attempt 2/DFIG1/rotor voltage equations ==
  w_e : Inport
  w_g : Inport  Port=2
  v_r : Inport  Port=3
  i_r : Inport  Port=4
  Complex to Real-Imag : ComplexToRealImag
  Divide : Product  Inputs=**
  Gain : Gain  Gain=R_r
  Gain1 : Gain  Gain=j
  Gain2 : Gain  Gain=314
  Integrator : Integrator
  Integrator1 : Integrator
  Real-Imag to Complex : RealImagToComplex
  Sum : Sum  Inputs=---
  Sum2 : Sum  Inputs=|+-
  f_r : Outport
  wires:
  Gain2/1 -> Gain1/1, f_r/1
  Gain1/1 -> Divide/2
  Complex to Real-Imag/2 -> Integrator1/1
  Complex to Real-Imag/1 -> Integrator/1
  Sum/1 -> Complex to Real-Imag/1
  w_g/1 -> Sum2/2
  w_e/1 -> Sum2/1
  Gain/1 -> Sum/1
  v_r/1 -> Sum/2
  i_r/1 -> Gain/1
  Real-Imag to Complex/1 -> Gain2/1
  Sum2/1 -> Divide/1
  Divide/1 -> Sum/3
  Integrator1/1 -> Real-Imag to Complex/2
  Integrator/1 -> Real-Imag to Complex/1

== system dfig_group_6_backsave/Attempt 2/DFIG1/stator voltage equations ==
  i_s : Inport
  v_s : Inport  Port=2
  w_e : Inport  Port=3
  Complex to Real-Imag : ComplexToRealImag
  Divide : Product  Inputs=**
  Gain : Gain  Gain=R_s
  Gain1 : Gain  Gain=j
  Gain2 : Gain  Gain=314
  Integrator : Integrator
  Integrator1 : Integrator
  Real-Imag to Complex : RealImagToComplex
  Sum : Sum  Inputs=---
  f_s : Outport
  wires:
  Gain2/1 -> Gain1/1, f_s/1
  Gain1/1 -> Divide/2
  Complex to Real-Imag/2 -> Integrator1/1
  Complex to Real-Imag/1 -> Integrator/1
  Sum/1 -> Complex to Real-Imag/1
  v_s/1 -> Sum/2
  Gain/1 -> Sum/1
  i_s/1 -> Gain/1
  Real-Imag to Complex/1 -> Gain2/1
  w_e/1 -> Divide/1
  Divide/1 -> Sum/3
  Integrator1/1 -> Real-Imag to Complex/2
  Integrator/1 -> Real-Imag to Complex/1

== system dfig_group_6_backsave/Subsystem/DFIG1/flux equations ==
  f_s : Inport
  f_r : Inport  Port=2
  Gain5 : Gain  Gain=1/L_s
  Gain7 : Gain  Gain=1/L_m
  Sum1 : Sum  Inputs=|+-
  Sum5 : Sum  Inputs=-+|
  i_s : Outport
  i_r : Outport  Port=2
  wires:
  Sum1/1 -> i_s/1
  Gain7/1 -> Sum1/1
  Sum5/1 -> Gain5/1
  f_r/1 -> Sum5/2
  Gain5/1 -> Sum1/2, i_r/1
  f_s/1 -> Sum5/1, Gain7/1

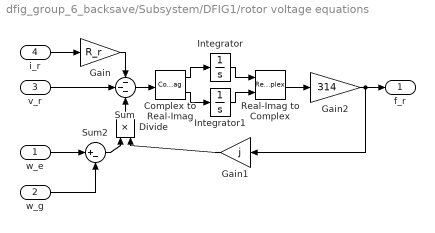
== system dfig_group_6_backsave/Subsystem/DFIG1/rotor voltage equations ==
  w_e : Inport
  w_g : Inport  Port=2
  v_r : Inport  Port=3
  i_r : Inport  Port=4
  Complex to Real-Imag : ComplexToRealImag
  Divide : Product  Inputs=**
  Gain : Gain  Gain=R_r
  Gain1 : Gain  Gain=j
  Gain2 : Gain  Gain=314
  Integrator : Integrator
  Integrator1 : Integrator
  Real-Imag to Complex : RealImagToComplex
  Sum : Sum  Inputs=---
  Sum2 : Sum  Inputs=|+-
  f_r : Outport
  wires:
  Gain2/1 -> Gain1/1, f_r/1
  Gain1/1 -> Divide/2
  Complex to Real-Imag/2 -> Integrator1/1
  Complex to Real-Imag/1 -> Integrator/1
  Sum/1 -> Complex to Real-Imag/1
  w_g/1 -> Sum2/2
  w_e/1 -> Sum2/1
  Gain/1 -> Sum/1
  v_r/1 -> Sum/2
  i_r/1 -> Gain/1
  Real-Imag to Complex/1 -> Gain2/1
  Sum2/1 -> Divide/1
  Divide/1 -> Sum/3
  Integrator1/1 -> Real-Imag to Complex/2
  Integrator/1 -> Real-Imag to Complex/1

== system dfig_group_6_backsave/Subsystem/DFIG1/stator voltage equations ==
  i_s : Inport
  v_s : Inport  Port=2
  w_e : Inport  Port=3
  Complex to Real-Imag : ComplexToRealImag
  Divide : Product  Inputs=**
  Gain : Gain  Gain=R_s
  Gain1 : Gain  Gain=j
  Gain2 : Gain  Gain=314
  Integrator : Integrator
  Integrator1 : Integrator
  Real-Imag to Complex : RealImagToComplex
  Sum : Sum  Inputs=---
  f_s : Outport
  wires:
  Gain2/1 -> Gain1/1, f_s/1
  Gain1/1 -> Divide/2
  Complex to Real-Imag/2 -> Integrator1/1
  Complex to Real-Imag/1 -> Integrator/1
  Sum/1 -> Complex to Real-Imag/1
  v_s/1 -> Sum/2
  Gain/1 -> Sum/1
  i_s/1 -> Gain/1
  Real-Imag to Complex/1 -> Gain2/1
  w_e/1 -> Divide/1
  Divide/1 -> Sum/3
  Integrator1/1 -> Real-Imag to Complex/2
  Integrator/1 -> Real-Imag to Complex/1

== system dfig_group_6_backsave/Subsystem1/DFIG1/flux equations ==
  f_s : Inport
  f_r : Inport  Port=2
  Gain5 : Gain  Gain=1/L_s
  Gain7 : Gain  Gain=1/L_m
  Sum1 : Sum  Inputs=|+-
  Sum5 : Sum  Inputs=-+|
  i_s : Outport
  i_r : Outport  Port=2
  wires:
  Sum1/1 -> i_s/1
  Gain7/1 -> Sum1/1
  Sum5/1 -> Gain5/1
  f_r/1 -> Sum5/2
  Gain5/1 -> Sum1/2, i_r/1
  f_s/1 -> Sum5/1, Gain7/1

== system dfig_group_6_backsave/Subsystem1/DFIG1/rotor voltage equations ==
  w_e : Inport
  w_g : Inport  Port=2
  v_r : Inport  Port=3
  i_r : Inport  Port=4
  Complex to Real-Imag : ComplexToRealImag
  Divide : Product  Inputs=**
  Gain : Gain  Gain=R_r
  Gain1 : Gain  Gain=j
  Gain2 : Gain  Gain=314
  Integrator : Integrator
  Integrator1 : Integrator
  Real-Imag to Complex : RealImagToComplex
  Sum : Sum  Inputs=---
  Sum2 : Sum  Inputs=|+-
  f_r : Outport
  wires:
  Gain2/1 -> Gain1/1, f_r/1
  Gain1/1 -> Divide/2
  Complex to Real-Imag/2 -> Integrator1/1
  Complex to Real-Imag/1 -> Integrator/1
  Sum/1 -> Complex to Real-Imag/1
  w_g/1 -> Sum2/2
  w_e/1 -> Sum2/1
  Gain/1 -> Sum/1
  v_r/1 -> Sum/2
  i_r/1 -> Gain/1
  Real-Imag to Complex/1 -> Gain2/1
  Sum2/1 -> Divide/1
  Divide/1 -> Sum/3
  Integrator1/1 -> Real-Imag to Complex/2
  Integrator/1 -> Real-Imag to Complex/1

== system dfig_group_6_backsave/Subsystem1/DFIG1/stator voltage equations ==
  i_s : Inport
  v_s : Inport  Port=2
  w_e : Inport  Port=3
  Complex to Real-Imag : ComplexToRealImag
  Divide : Product  Inputs=**
  Gain : Gain  Gain=R_s
  Gain1 : Gain  Gain=j
  Gain2 : Gain  Gain=314
  Integrator : Integrator
  Integrator1 : Integrator
  Real-Imag to Complex : RealImagToComplex
  Sum : Sum  Inputs=---
  f_s : Outport
  wires:
  Gain2/1 -> Gain1/1, f_s/1
  Gain1/1 -> Divide/2
  Complex to Real-Imag/2 -> Integrator1/1
  Complex to Real-Imag/1 -> Integrator/1
  Sum/1 -> Complex to Real-Imag/1
  v_s/1 -> Sum/2
  Gain/1 -> Sum/1
  i_s/1 -> Gain/1
  Real-Imag to Complex/1 -> Gain2/1
  w_e/1 -> Divide/1
  Divide/1 -> Sum/3
  Integrator1/1 -> Real-Imag to Complex/2
  Integrator/1 -> Real-Imag to Complex/1
